simulink subsystem "thermal"  (R2023b)
settings: Solver=VariableStepAuto  StartTime=0.0  StopTime=10.0  RelTol=1e-3
settings Model: Creator=gio  LastModifiedBy=gio

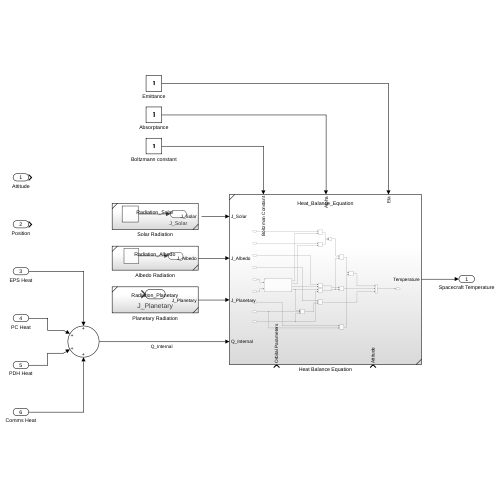
[thumbnail: Simulink's stored preview of the top-level diagram]
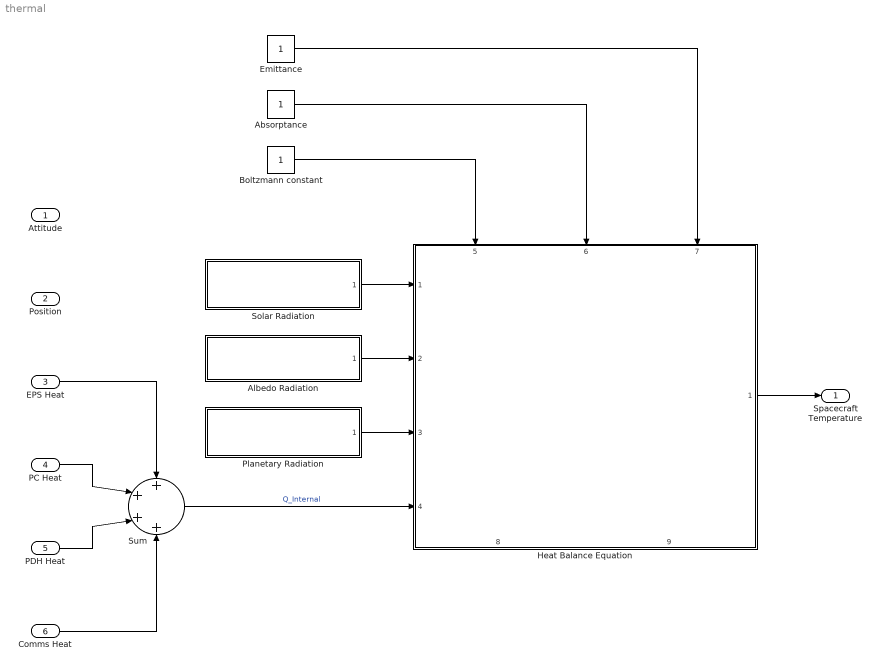
== system thermal ==
  Attitude : Inport
  Position : Inport  Port=2
  EPS Heat : Inport  Port=3
  PC Heat : Inport  Port=4
  PDH Heat : Inport  Port=5
  Comms Heat : Inport  Port=6
  Absorptance : Constant
  Albedo Radiation : Subsystem  ReferencedSubsystem=Radiation_Albedo
  Boltzmann constant : Constant
  Emittance : Constant
  Heat Balance Equation : Subsystem  ReferencedSubsystem=Heat_Balance_Equation
      settings: PortSchema="{\"entries\":[{\"content\":{\"sides\":[{\"content\":{\"connectorIds\":[\"In1\",\"In2\",\"In3\",\"In4\"]},\"type\":\"ConnectorPlacement.EquallySpacedRectSide\",\"uuid\":\"a25b9e7a-7ff8-41a7-9f1d-c6a99f23b8fe\"},{\"content\":{\"connectorIds\":[\"Out1\"],\"side\":\"RIGHT\"},\"type\":\"ConnectorPlacement.EquallySpacedRectSide\",\"uuid\":\"d83a7c11-be56-4082-830d-8ef9d7a83d1c\"},{\"content\":{\"connectorIds\":[\"In5\",\"In6\",\"In7\"],\"side\":\"TOP\"},\"type\":\"ConnectorPlacement.EquallySpacedRectSide\",\"uuid\":\"eb98d061-36e6-4e05-921e-b89c3305e4a0\"},{\"content\":{\"connectorIds\":[\"In8\",\"In9\"],\"side\":\"BOTTOM\"},\"type\":\"ConnectorPlacement.EquallySpacedRectSide\",\"uuid\":\"53606723-e8b3-4c8b-930e-9844b9467044\"}]},\"type\":\"ConnectorPlacement.EquallySpacedConnector\",\"uuid\":\"34fae694-3bd9-43d0-ade2-1fca4a12a03c\"}],\"packageUris\":[\"http://schema.mathworks.com/mf0/Connector/R2020b\"],\"version\":\"1.0\"}"
  Planetary Radiation : Subsystem  ReferencedSubsystem=Radiation_Planetary
  Solar Radiation : Subsystem  ReferencedSubsystem=Radiation_Solar
  Sum : Sum  Inputs=++++
  Spacecraft Temperature : Outport
  wires:
  EPS Heat/1 -> Sum/1
  PC Heat/1 -> Sum/2
  PDH Heat/1 -> Sum/3
  Comms Heat/1 -> Sum/4
  Sum/1 -> Heat Balance Equation/4  "Q_Internal"
  Absorptance/1 -> Heat Balance Equation/6
  Boltzmann constant/1 -> Heat Balance Equation/5
  Emittance/1 -> Heat Balance Equation/7
  Heat Balance Equation/1 -> Spacecraft Temperature/1
  Solar Radiation/1 -> Heat Balance Equation/1
  Albedo Radiation/1 -> Heat Balance Equation/2
  Planetary Radiation/1 -> Heat Balance Equation/3
